simulink model "project_bonus"  (R2012b)
settings: Solver=ode45  StartTime=0.0  StopTime=Inf  FixedStep=0.01  RelTol=1e-3
libraries: simulink x2
settings Model: ExtModeTrigDuration=5000  Creator=adith  LastModifiedBy=adith
settings SolverCC: PositivePriorityOrder=on
settings RTWCC: SystemTargetFile=quarc_win64.tlc  TemplateMakefile=quarc_default_tmf  Description=QUARC Win64 Target  ProcessScript=quarc_win64_make_rtw_hook
settings STFCustomTargetCC: TargetPreCompLibLocation=C:\PROGRA~3\QUARC\lib\2012b\win64\release  CodeReplacementLibrary=ANSI_C  GeneratePreprocessorConditionals=Disable all  CombineOutputUpdateFcns=on  GRTInterface=off  SystemTargetFile=quarc_win64.tlc
settings GRTTargetCC: TargetPreCompLibLocation=C:\PROGRA~3\QUARC\lib\2012b\win64\release  ParMdlRefBuildCompliant=off  CompOptLevelCompliant=off  ConcurrentExecutionCompliant=off  MatFileLogging=off  ExtMode=on  ExtModeMexFile=quarc_comm

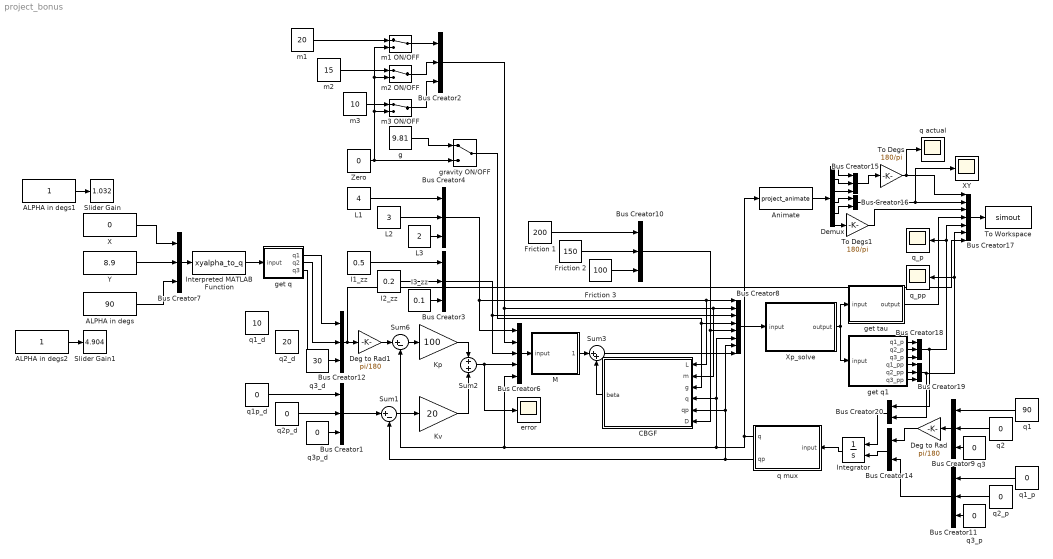
== system project_bonus ==
  ALPHA in degs : Constant  Value=90
  ALPHA in degs1 : Constant
  ALPHA in degs2 : Constant
  Animate : MATLABFcn  MATLABFcn=project_animate  OutputDimensions=6  OutputSignalType=real
  Bus Creator{1..4,7,9..12,15,18..19} (12 alike) : BusCreator  Inputs=3
  Bus Creator14 : BusCreator  Inputs=2
  Bus Creator16 : BusCreator  Inputs=2
  Bus Creator17 : BusCreator  Inputs=7
  Bus Creator20 : BusCreator  Inputs=2
  Bus Creator6 : BusCreator  Inputs=5
  Bus Creator8 : BusCreator  Inputs=8
  CBGF : MATLAB Function  TreatAsAtomicUnit=on
  Deg to Rad : Gain  Gain=pi/180
  Deg to Rad1 : Gain  Gain=pi/180
  Demux : Demux  Outputs=6
  Friction 1 : Constant  Value=200
  Friction 2 : Constant  Value=150
  Friction 3 : Constant  Value=100
  I1_zz : Constant  Value=0.5
  I2_zz : Constant  Value=0.2
  I3_zz : Constant  Value=0.1
  Integrator : Integrator  InitialConditionSource=external
  Interpreted MATLAB Function : MATLABFcn  MATLABFcn=xyalpha_to_q  OutputDimensions=3
  Kp : Gain  Gain=100
  Kv : Gain  Gain=20
  L1 : Constant  Value=4
  L2 : Constant  Value=3
  L3 : Constant  Value=2
  M : MATLAB Function  TreatAsAtomicUnit=on
  Slider Gain : simulink/Math Operations/Slider Gain  low=-4  gain=1.032  high=8.9
  Slider Gain1 : simulink/Math Operations/Slider Gain  low=3.5  gain=4.904  high=8.9
  Sum1 : Sum  Inputs=|+-
  Sum2 : Sum  Inputs=+|+
  Sum3 : Sum  Inputs=|++
  Sum6 : Sum  Inputs=|+-
  To Degs : Gain  Gain=180/pi
  To Degs1 : Gain  Gain=180/pi
  To Workspace : ToWorkspace  VariableName=simout  SampleTime=-1  SaveFormat=Structure With Time
  X : Constant  Value=0
  XY : Scope
      settings: ShowLegends=on  TimeRange=10  YMin=-8  YMax=9  SaveName=ScopeData4
  Xp_solve : MATLAB Function  TreatAsAtomicUnit=on
  Y : Constant  Value=8.9
  Zero : Constant  Value=0
  error : Scope
      settings: ShowLegends=on  TimeRange=8  YMin=-2.75  YMax=2.5  SaveName=ScopeData3
  g : Constant  Value=9.81
  get q : MATLAB Function  TreatAsAtomicUnit=on
  get q1 : MATLAB Function  TreatAsAtomicUnit=on
  get tau : MATLAB Function  TreatAsAtomicUnit=on
  gravity ON/OFF : ManualSwitch
  m1 : Constant  Value=20
  m1 ON/OFF : ManualSwitch
  m2 : Constant  Value=15
  m2 ON/OFF : ManualSwitch
  m3 : Constant  Value=10
  m3 ON/OFF : ManualSwitch
  q actual : Scope
      settings: ShowLegends=on  TimeRange=10  YMin=-100  YMax=175
  q mux : MATLAB Function  TreatAsAtomicUnit=on
  q1 : Constant  Value=90
  q1_d : Constant  Value=10
  q1_p : Constant  Value=0
  q1p_d : Constant  Value=0
  q2 : Constant  Value=0
  q2_d : Constant  Value=20
  q2_p : Constant  Value=0
  q2p_d : Constant  Value=0
  q3 : Constant  Value=0
  q3_d : Constant  Value=30
  q3_p : Constant  Value=0
  q3p_d : Constant  Value=0
  q_p : Scope
      settings: ShowLegends=on  TimeRange=20  YMin=-1.75  YMax=1.5
  q_pp : Scope
      settings: ShowLegends=on  TimeRange=20  YMin=-75  YMax=40  SaveName=ScopeData2
  wires:
  Bus Creator7/1 -> Interpreted MATLAB Function/1
  Interpreted MATLAB Function/1 -> get q/1(input)
  ALPHA in degs1/1 -> Slider Gain/1
  m1/1 -> m1 ON/OFF/1
  m3 ON/OFF/1 -> Bus Creator2/3
  m3/1 -> m3 ON/OFF/1
  m1 ON/OFF/1 -> Bus Creator2/1
  m2 ON/OFF/1 -> Bus Creator2/2
  m2/1 -> m2 ON/OFF/1
  Zero/1 -> m1 ON/OFF/2, m2 ON/OFF/2, m3 ON/OFF/2, gravity ON/OFF/2
  Friction 3/1 -> Bus Creator10/3
  Friction 2/1 -> Bus Creator10/2
  Friction 1/1 -> Bus Creator10/1
  g/1 -> gravity ON/OFF/1
  q1p_d/1 -> Bus Creator1/1
  q2p_d/1 -> Bus Creator1/2
  q3p_d/1 -> Bus Creator1/3
  I2_zz/1 -> Bus Creator3/2
  I3_zz/1 -> Bus Creator3/3
  L1/1 -> Bus Creator4/1
  L2/1 -> Bus Creator4/2
  L3/1 -> Bus Creator4/3
  Sum6/1 -> Kp/1
  Sum1/1 -> Kv/1
  Bus Creator1/1 -> Sum1/1
  Kp/1 -> Sum2/1
  Kv/1 -> Sum2/2
  Bus Creator4/1 -> CBGF/1(L), Bus Creator8/1, Bus Creator6/1
  Bus Creator2/1 -> CBGF/2(m), Bus Creator8/2, Bus Creator6/2
  Bus Creator3/1 -> Bus Creator6/3, Bus Creator8/3
  Sum2/1 -> error/1, Bus Creator6/4
  Bus Creator6/1 -> M/1(input)
  M/1(tau_wM) -> Sum3/1
  CBGF/1(beta) -> Sum3/2
  gravity ON/OFF/1 -> CBGF/3(g), Bus Creator8/4
  Bus Creator10/1 -> CBGF/6(D), Bus Creator8/5
  I1_zz/1 -> Bus Creator3/1
  Sum3/1 -> Bus Creator8/8
  Integrator/1 -> q mux/1(input)
  Bus Creator8/1 -> Xp_solve/1(input)
  q1/1 -> Bus Creator9/1
  q2/1 -> Bus Creator9/2
  q3/1 -> Bus Creator9/3
  q1_p/1 -> Bus Creator11/1
  q2_p/1 -> Bus Creator11/2
  q3_p/1 -> Bus Creator11/3
  Bus Creator11/1 -> Bus Creator14/2
  Bus Creator9/1 -> Deg to Rad/1
  Deg to Rad/1 -> Bus Creator14/1
  Bus Creator12/1 -> Bus Creator17/7, Deg to Rad1/1
  Deg to Rad1/1 -> Sum6/1
  q mux/1(q) -> Bus Creator8/6, CBGF/4(q), Bus Creator6/5, Sum6/2, Animate/1
  q mux/2(qp) -> Bus Creator8/7, CBGF/5(qp), Sum1/2
  Bus Creator17/1 -> To Workspace/1
  Animate/1 -> Demux/1
  Demux/1 -> Bus Creator15/1
  Demux/2 -> Bus Creator15/2
  Demux/3 -> Bus Creator15/3
  Bus Creator15/1 -> To Degs/1
  Demux/4 -> Bus Creator16/1
  Demux/5 -> Bus Creator16/2
  Demux/6 -> To Degs1/1
  To Degs/1 -> q actual/1, Bus Creator17/1
  Bus Creator16/1 -> XY/1, Bus Creator17/2
  To Degs1/1 -> Bus Creator17/3
  Xp_solve/1(output) -> get q1/1(input), get tau/1(input)
  get tau/1(output) -> Bus Creator17/4
  Bus Creator18/1 -> Bus Creator20/1, q_p/1, Bus Creator17/5
  Bus Creator19/1 -> Bus Creator20/2, q_pp/1, Bus Creator17/6
  Bus Creator20/1 -> Integrator/1
  get q1/1(q1_p) -> Bus Creator18/1
  get q1/2(q2_p) -> Bus Creator18/2
  get q1/3(q3_p) -> Bus Creator18/3
  get q1/4(q1_pp) -> Bus Creator19/1
  get q1/5(q2_pp) -> Bus Creator19/2
  get q1/6(q3_pp) -> Bus Creator19/3
  get q/1(q1) -> Bus Creator12/1
  get q/2(q2) -> Bus Creator12/2
  get q/3(q3) -> Bus Creator12/3
  Bus Creator14/1 -> Integrator/2
  ALPHA in degs2/1 -> Slider Gain1/1
  ALPHA in degs/1 -> Bus Creator7/3
  X/1 -> Bus Creator7/1
  Y/1 -> Bus Creator7/2

== matlab function project_bonus/M ==
  data: input input; tau_wM output
function tau_wM  = M_matrix(input)
    L1 = input(1);
    L2 = input(2);
    L3 = input(3);
    m1 = input(4);
    m2 = input(5);
    m3 = input(6);
    I1_zz = input(7);
    I2_zz = input(8);
    I3_zz = input(9);
    tau1 = input(10);
    tau2 = input(11);
    tau3 = input(12);
    q1 = input(13);
    q2 = input(14);
    q3 = input(15);
%     g = input(10);
%     D1 = input(11);
%     D2 = input(12);
%     D3 = input(13);
    tau_p = [tau1; tau2; tau3];
    M = [(I1_zz + I2_zz + I3_zz + (L1^2*m1)/4 + L1^2*m2 + L1^2*m3 + (L2^2*m2)/4 + L2^2*m3 + (L3^2*m3)/4 + L1*L3*m3*cos(q2 + q3) + L1*L2*m2*cos(q2) + 2*L1*L2*m3*cos(q2) + L2*L3*m3*cos(q3)), (I2_zz + I3_zz + (L2^2*m2)/4 + L2^2*m3 + (L3^2*m3)/4 + (L1*L3*m3*cos(q2 + q3))/2 + (L1*L2*m2*cos(q2))/2 + L1*L2*m3*cos(q2) + L2*L3*m3*cos(q3)), (I3_zz + (L3^2*m3)/4 + (L1*L3*m3*cos(q2 + q3))/2 + (L2*L3*m3*cos(q3))/2);
         (I2_zz + I3_zz + (L2^2*m2)/4 + L2^2*m3 + (L3^2*m3)/4 + (L1*L3*m3*cos(q2 + q3))/2 + (L1*L2*m2*cos(q2))/2 + L1*L2*m3*cos(q2) + L2*L3*m3*cos(q3)),                                                                       (I2_zz + I3_zz + (L2^2*m2)/4 + L2^2*m3 + (L3^2*m3)/4 + L2*L3*m3*cos(q3)),                             ((m3*L3^2)/4 + (L2*m3*cos(q3)*L3)/2 + I3_zz);
         (I3_zz + (L3^2*m3)/4 + (L1*L3*m3*cos(q2 + q3))/2 + (L2*L3*m3*cos(q3))/2),                                                                                                   ((m3*L3^2)/4 + (L2*m3*cos(q3)*L3)/2 + I3_zz),                                                    ((m3*L3^2)/4 + I3_zz)];
    tau_wM = M*tau_p;
end

== matlab function project_bonus/CBGF ==
  data: L input; beta output; m input; g input; q input; qp input; D input
function beta  = CBGF(L, m, g, q, qp, D)
    L1 = L(1);
    L2 = L(2);
    L3 = L(3);
    m1 = m(1);
    m2 = m(2);
    m3 = m(3);
    q1 = q(1);
    q2 = q(2);
    q3 = q(3);
    q1_p = qp(1);
    q2_p = qp(2);
    q3_p = qp(3);
    D1 = D(1);
    D2 = D(2);
    D3 = D(3);
        
%     g = input(10);
%     D1 = input(11);
%     D2 = input(12);
%     D3 = input(13);

    G =[((5*g*(7*L2*cos(q1 + q2) + 14*L1*cos(q1) + 2*L3*cos(q1 + q2 + q3)))/2);
                  (5*L3*g*cos(q1 + q2 + q3) + (35*L2*g*cos(q1 + q2))/2);
                                             (5*L3*g*cos(q1 + q2 + q3))]; 
    F = [D1*q1_p;
        D2*q2_p;
        D3*q3_p];
    B = [ (-L1*(L3*m3*sin(q2 + q3) + L2*m2*sin(q2) + 2*L2*m3*sin(q2))), (-L3*m3*(L1*sin(q2 + q3) + L2*sin(q3))), (-L3*m3*(L1*sin(q2 + q3) + L2*sin(q3)));
                                                          0,                     (-L2*L3*m3*sin(q3)),                     (-L2*L3*m3*sin(q3));
                                           (L2*L3*m3*sin(q3)),                                     0,                                     0];

    C =[                                                             0, (-(L1*(L3*m3*sin(q2 + q3) + L2*m2*sin(q2) + 2*L2*m3*sin(q2)))/2), (-(L3*m3*(L1*sin(q2 + q3) + L2*sin(q3)))/2);
         ((L1*(L3*m3*sin(q2 + q3) + L2*m2*sin(q2) + 2*L2*m3*sin(q2)))/2),                                                              0,                     (-(L2*L3*m3*sin(q3))/2);
                              ((L3*m3*(L1*sin(q2 + q3) + L2*sin(q3)))/2),                                           ((L2*L3*m3*sin(q3))/2),                                         0];
    V =  C*[q1_p^2; q2_p^2; q3_p^2] + B*[q1_p*q2_p; q1_p*q3_p; q2_p*q3_p];
    beta = V + G + F;
end

== matlab function project_bonus/get tau ==
  data: input input; output output
function output  = get_tau(input)
    tau1 = input(7);
    tau2 = input(8);
    tau3 = input(9);
    output = [tau1, tau2, tau3];
end

== matlab function project_bonus/get q ==
  data: input input; q1 output; q2 output; q3 output
function [q1, q2, q3]  = get_q(input)
    q1 = input(1);
    q2 = input(2);
    q3 = input(3);
%     q1 = atan2(sin(q1),cos(q1));
%     q2 = atan2(sin(q2),cos(q2));
%     q3 = atan2(sin(q3),cos(q3));
    %output = [q1, q2, q3, q1_p, q2_p, q3_p];
end

== matlab function project_bonus/get q1 ==
  data: input input; q1_p output; q2_p output; q3_p output; q1_pp output; q2_pp output; q3_pp output
function [q1_p, q2_p, q3_p, q1_pp, q2_pp, q3_pp]  = get_q(input)
    q1_p = input(1);
    q2_p = input(2);
    q3_p = input(3);
    q1_pp = input(4);
    q2_pp = input(5);
    q3_pp = input(6);
    %output = [q1_p, q2_p, q3_p, q1_pp, q2_pp, q3_pp];
end

== matlab function project_bonus/Xp_solve ==
  data: input input; output output
function output  = Xp_solve(input)
    L1 = input(1);
    L2 = input(2);
    L3 = input(3);
    m1 = input(4);
    m2 = input(5);
    m3 = input(6);
    I1_zz = input(7);
    I2_zz = input(8);
    I3_zz = input(9);
    g = input(10);
    D1 = input(11);
    D2 = input(12);
    D3 = input(13);
    q1 = input(14);
    q2 = input(15);
    q3 = input(16);
    q1_p = input(17);
    q2_p = input(18);
    q3_p = input(19);
    tau1 = input(20);
    tau2 = input(21);
    tau3 = input(22);
    q1_pp = (2*(32*I2_zz*I3_zz*tau1 - 32*I2_zz*I3_zz*tau2 + 8*I3_zz*L2^2*m2*tau1 + 8*I2_zz*L3^2*m3*tau1 - 8*I3_zz*L2^2*m2*tau2 + 32*I3_zz*L2^2*m3*tau1 - 8*I2_zz*L3^2*m3*tau2 - 32*I3_zz*L2^2*m3*tau2 - 32*D1*I2_zz*I3_zz*q1_p + 32*D2*I2_zz*I3_zz*q2_p + 4*L2^2*L3^2*m3^2*tau1 - 4*L2^2*L3^2*m3^2*tau2 + 2*L2^2*L3^2*m2*m3*tau1 - 2*L2^2*L3^2*m2*m3*tau2 - 4*L2^2*L3^2*m3^2*tau1*cos(2*q3) + 4*L2^2*L3^2*m3^2*tau2*cos(2*q3) - 4*D1*L2^2*L3^2*m3^2*q1_p + 4*D2*L2^2*L3^2*m3^2*q2_p - 8*D1*I3_zz*L2^2*m2*q1_p - 8*D1*I2_zz*L3^2*m3*q1_p - 32*D1*I3_zz*L2^2*m3*q1_p + 8*D2*I3_zz*L2^2*m2*q2_p + 8*D2*I2_zz*L3^2*m3*q2_p + 32*D2*I3_zz*L2^2*m3*q2_p - 1120*I2_zz*I3_zz*L1*g*cos(q1) - 85*L1*L2^2*L3^2*g*m3^2*cos(q1) - 15*L1*L2^2*L3^2*g*m3^2*cos(q1 + 2*q2 + 2*q3) + 4*I2_zz*L1^2*L3^2*m3^2*q1_p^2*sin(2*q2 + 2*q3) + 4*I3_zz*L1*L2^3*m2^2*q1_p^2*sin(q2) + 4*I3_zz*L1*L2^3*m2^2*q2_p^2*sin(q2) + 32*I3_zz*L1*L2^3*m3^2*q1_p^2*sin(q2) + 32*I3_zz*L1*L2^3*m3^2*q2_p^2*sin(q2) + 15*L1*L2^2*L3^2*g*m3^2*cos(q1 + 2*q2) + 35*L1*L2^2*L3^2*g*m3^2*cos(q1 - 2*q3) + 50*L1*L2^2*L3^2*g*m3^2*cos(q1 + 2*q3) - 2*D1*L2^2*L3^2*m2*m3*q1_p + 2*D2*L2^2*L3^2*m2*m3*q2_p - 140*I3_zz*L1*L2^2*g*m2*cos(q1) - 240*I2_zz*L1*L3^2*g*m3*cos(q1) - 840*I3_zz*L1*L2^2*g*m3*cos(q1) + 40*I2_zz*L1*L3^2*g*m3*cos(q1 + 2*q2 + 2*q3) + 4*D1*L2^2*L3^2*m3^2*q1_p*cos(2*q3) - 4*D2*L2^2*L3^2*m3^2*q2_p*cos(2*q3) + 140*I3_zz*L1*L2^2*g*m2*cos(q1 + 2*q2) + 280*I3_zz*L1*L2^2*g*m3*cos(q1 + 2*q2) - 8*L1*L2^2*L3*m3^2*tau3*cos(q2 + q3) - 4*L1*L2*L3^2*m3^2*tau2*cos(q2) + 4*L1*L2*L3^2*m3^2*tau3*cos(q2) - 16*I2_zz*L1*L3*m3*tau3*cos(q2 + q3) + 4*I3_zz*L1^2*L2^2*m2^2*q1_p^2*sin(2*q2) + 16*I3_zz*L1^2*L2^2*m3^2*q1_p^2*sin(2*q2) + 4*L1*L2*L3^2*m3^2*tau2*cos(q2 + 2*q3) + 8*L1*L2^2*L3*m3^2*tau3*cos(q2 - q3) - 4*L1*L2*L3^2*m3^2*tau3*cos(q2 + 2*q3) + 4*I2_zz*L1*L3^3*m3^2*q1_p^2*sin(q2 + q3) + 4*I2_zz*L1*L3^3*m3^2*q2_p^2*sin(q2 + q3) + 4*I2_zz*L1*L3^3*m3^2*q3_p^2*sin(q2 + q3) - 16*I3_zz*L1*L2*m2*tau2*cos(q2) + 16*I3_zz*L1*L2*m2*tau3*cos(q2) - 32*I3_zz*L1*L2*m3*tau2*cos(q2) + 32*I3_zz*L1*L2*m3*tau3*cos(q2) + 8*I2_zz*L1*L3^3*m3^2*q1_p*q2_p*sin(q2 + q3) + 8*I2_zz*L1*L3^3*m3^2*q1_p*q3_p*sin(q2 + q3) + 8*I2_zz*L1*L3^3*m3^2*q2_p*q3_p*sin(q2 + q3) + 16*D3*I2_zz*L1*L3*m3*q3_p*cos(q2 + q3) - 35*L1*L2^2*L3^2*g*m2*m3*cos(q1) + L1*L2^2*L3^3*m2*m3^2*q1_p^2*sin(q2 - q3) + L1*L2^2*L3^3*m2*m3^2*q2_p^2*sin(q2 - q3) - L1*L2^3*L3^2*m2*m3^2*q1_p^2*sin(q2 + 2*q3) + L1*L2^2*L3^3*m2*m3^2*q3_p^2*sin(q2 - q3) - L1*L2^3*L3^2*m2*m3^2*q2_p^2*sin(q2 + 2*q3) - 4*D2*L1*L2*L3^2*m3^2*q2_p*cos(q2 + 2*q3) - 8*D3*L1*L2^2*L3*m3^2*q3_p*cos(q2 - q3) + 4*D3*L1*L2*L3^2*m3^2*q3_p*cos(q2 + 2*q3) + 24*I3_zz*L1*L2^3*m2*m3*q1_p^2*sin(q2) + 24*I3_zz*L1*L2^3*m2*m3*q2_p^2*sin(q2) + 8*I3_zz*L1*L2^3*m2^2*q1_p*q2_p*sin(q2) + 64*I3_zz*L1*L2^3*m3^2*q1_p*q2_p*sin(q2) + 16*D2*I3_zz*L1*L2*m2*q2_p*cos(q2) + 32*D2*I3_zz*L1*L2*m3*q2_p*cos(q2) - 16*D3*I3_zz*L1*L2*m2*q3_p*cos(q2) - 32*D3*I3_zz*L1*L2*m3*q3_p*cos(q2) + 8*I3_zz*L1*L2^2*L3*m3^2*q1_p^2*sin(q2 + q3) + 8*I3_zz*L1*L2^2*L3*m3^2*q2_p^2*sin(q2 + q3) + 8*I3_zz*L1*L2^2*L3*m3^2*q3_p^2*sin(q2 + q3) + 25*L1*L2^2*L3^2*g*m2*m3*cos(q1 + 2*q2) - 10*L1*L2^2*L3^2*g*m2*m3*cos(q1 + 2*q3) + 4*I2_zz*L1*L2*L3^2*m3^2*q1_p^2*sin(q2) + 4*I2_zz*L1*L2*L3^2*m3^2*q2_p^2*sin(q2) + 16*I2_zz*I3_zz*L1*L3*m3*q1_p^2*sin(q2 + q3) + 16*I2_zz*I3_zz*L1*L3*m3*q2_p^2*sin(q2 + q3) + 16*I2_zz*I3_zz*L1*L3*m3*q3_p^2*sin(q2 + q3) + 4*I2_zz*L1*L2*L3^2*m3^2*q1_p^2*sin(q2 + 2*q3) + 8*I3_zz*L1*L2^2*L3*m3^2*q1_p^2*sin(q2 - q3) + 4*I2_zz*L1*L2*L3^2*m3^2*q2_p^2*sin(q2 + 2*q3) + 8*I3_zz*L1*L2^2*L3*m3^2*q2_p^2*sin(q2 - q3) + 8*I3_zz*L1*L2^2*L3*m3^2*q3_p^2*sin(q2 - q3) + 16*I2_zz*I3_zz*L1*L2*m2*q1_p^2*sin(q2) + 16*I2_zz*I3_zz*L1*L2*m2*q2_p^2*sin(q2) + 32*I2_zz*I3_zz*L1*L2*m3*q1_p^2*sin(q2) + 32*I2_zz*I3_zz*L1*L2*m3*q2_p^2*sin(q2) + 2*L1^2*L2^2*L3^2*m2*m3^2*q1_p^2*sin(2*q2) + L1^2*L2^2*L3^2*m2^2*m3*q1_p^2*sin(2*q2) - 4*L1*L2*L3^2*m2*m3*tau2*cos(q2) + 4*L1*L2*L3^2*m2*m3*tau3*cos(q2) + 8*D3*L1*L2^2*L3*m3^2*q3_p*cos(q2 + q3) - L1^2*L2^2*L3^2*m2*m3^2*q1_p^2*sin(2*q2 + 2*q3) + 16*I3_zz*L1^2*L2^2*m2*m3*q1_p^2*sin(2*q2) + 3*L1*L2^3*L3^2*m2*m3^2*q1_p^2*sin(q2) + L1*L2^3*L3^2*m2^2*m3*q1_p^2*sin(q2) + 3*L1*L2^3*L3^2*m2*m3^2*q2_p^2*sin(q2) + L1*L2^3*L3^2*m2^2*m3*q2_p^2*sin(q2) + 4*L1*L2^2*L3*m2*m3*tau3*cos(q2 - q3) + 4*D2*L1*L2*L3^2*m3^2*q2_p*cos(q2) - 4*D3*L1*L2*L3^2*m3^2*q3_p*cos(q2) + 6*L1*L2^3*L3^2*m2*m3^2*q1_p*q2_p*sin(q2) + 2*L1*L2^3*L3^2*m2^2*m3*q1_p*q2_p*sin(q2) + 4*D2*L1*L2*L3^2*m2*m3*q2_p*cos(q2) - 4*D3*L1*L2*L3^2*m2*m3*q3_p*cos(q2) + 2*L1*L2^2*L3^3*m2*m3^2*q1_p*q2_p*sin(q2 - q3) + 2*L1*L2^2*L3^3*m2*m3^2*q1_p*q3_p*sin(q2 - q3) - 2*L1*L2^3*L3^2*m2*m3^2*q1_p*q2_p*sin(q2 + 2*q3) + 2*L1*L2^2*L3^3*m2*m3^2*q2_p*q3_p*sin(q2 - q3) - 4*D3*L1*L2^2*L3*m2*m3*q3_p*cos(q2 - q3) + 48*I3_zz*L1*L2^3*m2*m3*q1_p*q2_p*sin(q2) + 16*I3_zz*L1*L2^2*L3*m3^2*q1_p*q2_p*sin(q2 + q3) + 16*I3_zz*L1*L2^2*L3*m3^2*q1_p*q3_p*sin(q2 + q3) + 16*I3_zz*L1*L2^2*L3*m3^2*q2_p*q3_p*sin(q2 + q3) + 4*I2_zz*L1*L2*L3^2*m2*m3*q1_p^2*sin(q2) + 4*I2_zz*L1*L2*L3^2*m2*m3*q2_p^2*sin(q2) + 8*I2_zz*L1*L2*L3^2*m3^2*q1_p*q2_p*sin(q2) + 32*I2_zz*I3_zz*L1*L3*m3*q1_p*q2_p*sin(q2 + q3) + 32*I2_zz*I3_zz*L1*L3*m3*q1_p*q3_p*sin(q2 + q3) + 32*I2_zz*I3_zz*L1*L3*m3*q2_p*q3_p*sin(q2 + q3) + 4*I3_zz*L1*L2^2*L3*m2*m3*q1_p^2*sin(q2 - q3) + 4*I3_zz*L1*L2^2*L3*m2*m3*q2_p^2*sin(q2 - q3) + 4*I3_zz*L1*L2^2*L3*m2*m3*q3_p^2*sin(q2 - q3) + 8*I2_zz*L1*L2*L3^2*m3^2*q1_p*q2_p*sin(q2 + 2*q3) + 16*I3_zz*L1*L2^2*L3*m3^2*q1_p*q2_p*sin(q2 - q3) + 16*I3_zz*L1*L2^2*L3*m3^2*q1_p*q3_p*sin(q2 - q3) + 16*I3_zz*L1*L2^2*L3*m3^2*q2_p*q3_p*sin(q2 - q3) + 32*I2_zz*I3_zz*L1*L2*m2*q1_p*q2_p*sin(q2) + 64*I2_zz*I3_zz*L1*L2*m3*q1_p*q2_p*sin(q2) + 8*I2_zz*L1*L2*L3^2*m2*m3*q1_p*q2_p*sin(q2) + 8*I3_zz*L1*L2^2*L3*m2*m3*q1_p*q2_p*sin(q2 - q3) + 8*I3_zz*L1*L2^2*L3*m2*m3*q1_p*q3_p*sin(q2 - q3) + 8*I3_zz*L1*L2^2*L3*m2*m3*q2_p*q3_p*sin(q2 - q3)))/(64*I1_zz*I2_zz*I3_zz + 16*I2_zz*I3_zz*L1^2*m1 + 16*I1_zz*I3_zz*L2^2*m2 + 64*I2_zz*I3_zz*L1^2*m2 + 16*I1_zz*I2_zz*L3^2*m3 + 64*I1_zz*I3_zz*L2^2*m3 + 64*I2_zz*I3_zz*L1^2*m3 + 8*I3_zz*L1^2*L2^2*m2^2 + 8*I1_zz*L2^2*L3^2*m3^2 + 8*I2_zz*L1^2*L3^2*m3^2 + 32*I3_zz*L1^2*L2^2*m3^2 - 8*I2_zz*L1^2*L3^2*m3^2*cos(2*q2 + 2*q3) + 2*L1^2*L2^2*L3^2*m1*m3^2 + 6*L1^2*L2^2*L3^2*m2*m3^2 + 2*L1^2*L2^2*L3^2*m2^2*m3 + 4*I3_zz*L1^2*L2^2*m1*m2 + 4*I2_zz*L1^2*L3^2*m1*m3 + 16*I3_zz*L1^2*L2^2*m1*m3 + 4*I1_zz*L2^2*L3^2*m2*m3 + 16*I2_zz*L1^2*L3^2*m2*m3 + 48*I3_zz*L1^2*L2^2*m2*m3 - 8*I3_zz*L1^2*L2^2*m2^2*cos(2*q2) - 32*I3_zz*L1^2*L2^2*m3^2*cos(2*q2) - 8*I1_zz*L2^2*L3^2*m3^2*cos(2*q3) - 32*I3_zz*L1^2*L2^2*m2*m3*cos(2*q2) + L1^2*L2^2*L3^2*m1*m2*m3 - 2*L1^2*L2^2*L3^2*m1*m3^2*cos(2*q3) - 4*L1^2*L2^2*L3^2*m2*m3^2*cos(2*q2) - 2*L1^2*L2^2*L3^2*m2^2*m3*cos(2*q2) - 4*L1^2*L2^2*L3^2*m2*m3^2*cos(2*q3) + 2*L1^2*L2^2*L3^2*m2*m3^2*cos(2*q2 + 2*q3)); 
    q2_pp = -(2*(32*I2_zz*I3_zz*tau1 - 32*I1_zz*I3_zz*tau2 + 32*I1_zz*I3_zz*tau3 - 32*I2_zz*I3_zz*tau2 - 8*I3_zz*L1^2*m1*tau2 + 8*I3_zz*L1^2*m1*tau3 - 32*I3_zz*L1^2*m2*tau2 + 8*I3_zz*L2^2*m2*tau1 - 8*I1_zz*L3^2*m3*tau2 + 8*I2_zz*L3^2*m3*tau1 + 32*I3_zz*L1^2*m2*tau3 - 32*I3_zz*L1^2*m3*tau2 - 8*I3_zz*L2^2*m2*tau2 + 32*I3_zz*L2^2*m3*tau1 + 8*I1_zz*L3^2*m3*tau3 - 8*I2_zz*L3^2*m3*tau2 + 32*I3_zz*L1^2*m3*tau3 - 32*I3_zz*L2^2*m3*tau2 - 32*D1*I2_zz*I3_zz*q1_p + 32*D2*I1_zz*I3_zz*q2_p + 32*D2*I2_zz*I3_zz*q2_p - 32*D3*I1_zz*I3_zz*q3_p - 4*L1^2*L3^2*m3^2*tau2 + 4*L2^2*L3^2*m3^2*tau1 + 4*L1^2*L3^2*m3^2*tau3 - 4*L2^2*L3^2*m3^2*tau2 - 2*L1^2*L3^2*m1*m3*tau2 + 2*L1^2*L3^2*m1*m3*tau3 - 8*L1^2*L3^2*m2*m3*tau2 + 2*L2^2*L3^2*m2*m3*tau1 + 8*L1^2*L3^2*m2*m3*tau3 - 2*L2^2*L3^2*m2*m3*tau2 - 4*L2^2*L3^2*m3^2*tau1*cos(2*q3) + 4*L2^2*L3^2*m3^2*tau2*cos(2*q3) - 4*D1*L2^2*L3^2*m3^2*q1_p + 4*D2*L1^2*L3^2*m3^2*q2_p + 4*D2*L2^2*L3^2*m3^2*q2_p - 4*D3*L1^2*L3^2*m3^2*q3_p + 560*I1_zz*I3_zz*L2*g*cos(q1 + q2) + 4*L1^2*L3^2*m3^2*tau2*cos(2*q2 + 2*q3) - 4*L1^2*L3^2*m3^2*tau3*cos(2*q2 + 2*q3) - 8*D1*I3_zz*L2^2*m2*q1_p + 8*D2*I3_zz*L1^2*m1*q2_p - 8*D1*I2_zz*L3^2*m3*q1_p - 32*D1*I3_zz*L2^2*m3*q1_p + 32*D2*I3_zz*L1^2*m2*q2_p + 8*D2*I1_zz*L3^2*m3*q2_p + 32*D2*I3_zz*L1^2*m3*q2_p + 8*D2*I3_zz*L2^2*m2*q2_p - 8*D3*I3_zz*L1^2*m1*q3_p + 8*D2*I2_zz*L3^2*m3*q2_p + 32*D2*I3_zz*L2^2*m3*q2_p - 32*D3*I3_zz*L1^2*m2*q3_p - 8*D3*I1_zz*L3^2*m3*q3_p - 32*D3*I3_zz*L1^2*m3*q3_p - 1120*I2_zz*I3_zz*L1*g*cos(q1) - 85*L1*L2^2*L3^2*g*m3^2*cos(q1) + 35*L1^2*L2*L3^2*g*m3^2*cos(q1 - q2 - 2*q3) - 15*L1*L2^2*L3^2*g*m3^2*cos(q1 + 2*q2 + 2*q3) - 15*L1^2*L2*L3^2*g*m3^2*cos(q1 + 3*q2 + 2*q3) + 4*I2_zz*L1^2*L3^2*m3^2*q1_p^2*sin(2*q2 + 2*q3) + 140*I3_zz*L1^2*L2*g*m1*cos(q1 + q2) + 280*I3_zz*L1^2*L2*g*m2*cos(q1 + q2) + 100*I1_zz*L2*L3^2*g*m3*cos(q1 + q2) + 4*I3_zz*L1*L2^3*m2^2*q1_p^2*sin(q2) + 16*I3_zz*L1^3*L2*m2^2*q1_p^2*sin(q2) + 4*I3_zz*L1*L2^3*m2^2*q2_p^2*sin(q2) + 32*I3_zz*L1*L2^3*m3^2*q1_p^2*sin(q2) + 32*I3_zz*L1^3*L2*m3^2*q1_p^2*sin(q2) - 4*I1_zz*L2*L3^3*m3^2*q1_p^2*sin(q3) + 32*I3_zz*L1*L2^3*m3^2*q2_p^2*sin(q2) - 4*I1_zz*L2*L3^3*m3^2*q2_p^2*sin(q3) - 4*I1_zz*L2*L3^3*m3^2*q3_p^2*sin(q3) - 50*L1^2*L2*L3^2*g*m3^2*cos(q1 - q2) + 15*L1*L2^2*L3^2*g*m3^2*cos(q1 + 2*q2) + 35*L1*L2^2*L3^2*g*m3^2*cos(q1 - 2*q3) + 50*L1*L2^2*L3^2*g*m3^2*cos(q1 + 2*q3) - 2*D1*L2^2*L3^2*m2*m3*q1_p + 2*D2*L1^2*L3^2*m1*m3*q2_p + 8*D2*L1^2*L3^2*m2*m3*q2_p + 2*D2*L2^2*L3^2*m2*m3*q2_p - 2*D3*L1^2*L3^2*m1*m3*q3_p - 8*D3*L1^2*L3^2*m2*m3*q3_p - 140*I3_zz*L1*L2^2*g*m2*cos(q1) - 240*I2_zz*L1*L3^2*g*m3*cos(q1) - 840*I3_zz*L1*L2^2*g*m3*cos(q1) + 40*I2_zz*L1*L3^2*g*m3*cos(q1 + 2*q2 + 2*q3) + 4*D1*L2^2*L3^2*m3^2*q1_p*cos(2*q3) - 4*D2*L2^2*L3^2*m3^2*q2_p*cos(2*q3) - 280*I3_zz*L1^2*L2*g*m2*cos(q1 - q2) + 140*I3_zz*L1*L2^2*g*m2*cos(q1 + 2*q2) - 560*I3_zz*L1^2*L2*g*m3*cos(q1 - q2) + 280*I3_zz*L1*L2^2*g*m3*cos(q1 + 2*q2) - 8*L1*L2^2*L3*m3^2*tau3*cos(q2 + q3) - 4*D2*L1^2*L3^2*m3^2*q2_p*cos(2*q2 + 2*q3) + 4*D3*L1^2*L3^2*m3^2*q3_p*cos(2*q2 + 2*q3) + 50*L1^2*L2*L3^2*g*m3^2*cos(q1 + q2 + 2*q3) + 4*L1*L2*L3^2*m3^2*tau1*cos(q2) - 8*L1*L2*L3^2*m3^2*tau2*cos(q2) + 4*L1*L2*L3^2*m3^2*tau3*cos(q2) + 8*L1^2*L2*L3*m3^2*tau3*cos(q3) - 16*I2_zz*L1*L3*m3*tau3*cos(q2 + q3) - 20*L1^2*L2*L3^2*g*m3^2*cos(q1 + q2) + 8*I3_zz*L1^2*L2^2*m2^2*q1_p^2*sin(2*q2) + 4*I3_zz*L1^2*L2^2*m2^2*q2_p^2*sin(2*q2) + 32*I3_zz*L1^2*L2^2*m3^2*q1_p^2*sin(2*q2) - 4*I1_zz*L2^2*L3^2*m3^2*q1_p^2*sin(2*q3) + 16*I3_zz*L1^2*L2^2*m3^2*q2_p^2*sin(2*q2) - 4*I1_zz*L2^2*L3^2*m3^2*q2_p^2*sin(2*q3) - 4*L1*L2*L3^2*m3^2*tau1*cos(q2 + 2*q3) + 8*L1*L2*L3^2*m3^2*tau2*cos(q2 + 2*q3) + 8*L1*L2^2*L3*m3^2*tau3*cos(q2 - q3) - 4*L1*L2*L3^2*m3^2*tau3*cos(q2 + 2*q3) - 8*L1^2*L2*L3*m3^2*tau3*cos(2*q2 + q3) - 40*I1_zz*L2*L3^2*g*m3*cos(q1 + q2 + 2*q3) + 4*I2_zz*L1*L3^3*m3^2*q1_p^2*sin(q2 + q3) + 4*I2_zz*L1*L3^3*m3^2*q2_p^2*sin(q2 + q3) + 4*I2_zz*L1*L3^3*m3^2*q3_p^2*sin(q2 + q3) + 16*I3_zz*L1*L2*m2*tau1*cos(q2) - 32*I3_zz*L1*L2*m2*tau2*cos(q2) + 32*I3_zz*L1*L2*m3*tau1*cos(q2) + 16*I3_zz*L1*L2*m2*tau3*cos(q2) - 64*I3_zz*L1*L2*m3*tau2*cos(q2) + 32*I3_zz*L1*L2*m3*tau3*cos(q2) + 16*I1_zz*L2*L3*m3*tau3*cos(q3) + 8*I2_zz*L1*L3^3*m3^2*q1_p*q2_p*sin(q2 + q3) + 8*I2_zz*L1*L3^3*m3^2*q1_p*q3_p*sin(q2 + q3) + 8*I2_zz*L1*L3^3*m3^2*q2_p*q3_p*sin(q2 + q3) + 16*D3*I2_zz*L1*L3*m3*q3_p*cos(q2 + q3) - 35*L1*L2^2*L3^2*g*m2*m3*cos(q1) + 10*L1^2*L2*L3^2*g*m2*m3*cos(q1 + 3*q2 + 2*q3) + L1*L2^2*L3^3*m2*m3^2*q1_p^2*sin(q2 - q3) - L1^3*L2*L3^2*m1*m3^2*q1_p^2*sin(q2 + 2*q3) + L1*L2^2*L3^3*m2*m3^2*q2_p^2*sin(q2 - q3) - L1*L2^3*L3^2*m2*m3^2*q1_p^2*sin(q2 + 2*q3) + L1^2*L2*L3^3*m2*m3^2*q1_p^2*sin(2*q2 + q3) - 2*L1^3*L2*L3^2*m2*m3^2*q1_p^2*sin(q2 + 2*q3) + L1*L2^2*L3^3*m2*m3^2*q3_p^2*sin(q2 - q3) - L1*L2^3*L3^2*m2*m3^2*q2_p^2*sin(q2 + 2*q3) + L1^2*L2*L3^3*m2*m3^2*q2_p^2*sin(2*q2 + q3) + L1^2*L2*L3^3*m2*m3^2*q3_p^2*sin(2*q2 + q3) + 4*D1*L1*L2*L3^2*m3^2*q1_p*cos(q2 + 2*q3) - 8*D2*L1*L2*L3^2*m3^2*q2_p*cos(q2 + 2*q3) - 8*D3*L1*L2^2*L3*m3^2*q3_p*cos(q2 - q3) + 4*D3*L1*L2*L3^2*m3^2*q3_p*cos(q2 + 2*q3) + 8*D3*L1^2*L2*L3*m3^2*q3_p*cos(2*q2 + q3) + 4*I3_zz*L1^3*L2*m1*m2*q1_p^2*sin(q2) + 8*I3_zz*L1^3*L2*m1*m3*q1_p^2*sin(q2) + 24*I3_zz*L1*L2^3*m2*m3*q1_p^2*sin(q2) + 48*I3_zz*L1^3*L2*m2*m3*q1_p^2*sin(q2) + 24*I3_zz*L1*L2^3*m2*m3*q2_p^2*sin(q2) + 8*I3_zz*L1*L2^3*m2^2*q1_p*q2_p*sin(q2) + 64*I3_zz*L1*L2^3*m3^2*q1_p*q2_p*sin(q2) - 8*I1_zz*L2*L3^3*m3^2*q1_p*q2_p*sin(q3) - 8*I1_zz*L2*L3^3*m3^2*q1_p*q3_p*sin(q3) - 8*I1_zz*L2*L3^3*m3^2*q2_p*q3_p*sin(q3) - 16*D1*I3_zz*L1*L2*m2*q1_p*cos(q2) - 32*D1*I3_zz*L1*L2*m3*q1_p*cos(q2) + 32*D2*I3_zz*L1*L2*m2*q2_p*cos(q2) + 64*D2*I3_zz*L1*L2*m3*q2_p*cos(q2) - 16*D3*I3_zz*L1*L2*m2*q3_p*cos(q2) - 32*D3*I3_zz*L1*L2*m3*q3_p*cos(q2) - 16*D3*I1_zz*L2*L3*m3*q3_p*cos(q3) + 8*I3_zz*L1*L2^2*L3*m3^2*q1_p^2*sin(q2 + q3) + 8*I3_zz*L1*L2^2*L3*m3^2*q2_p^2*sin(q2 + q3) + 8*I3_zz*L1*L2^2*L3*m3^2*q3_p^2*sin(q2 + q3) - 60*L1^2*L2*L3^2*g*m2*m3*cos(q1 - q2) + 25*L1*L2^2*L3^2*g*m2*m3*cos(q1 + 2*q2) - 10*L1*L2^2*L3^2*g*m2*m3*cos(q1 + 2*q3) + 4*I1_zz*L1*L2*L3^2*m3^2*q1_p^2*sin(q2) + 4*I2_zz*L1*L2*L3^2*m3^2*q1_p^2*sin(q2) + 4*I2_zz*L1*L2*L3^2*m3^2*q2_p^2*sin(q2) - 8*I3_zz*L1^2*L2*L3*m3^2*q1_p^2*sin(q3) - 8*I3_zz*L1^2*L2*L3*m3^2*q2_p^2*sin(q3) - 8*I3_zz*L1^2*L2*L3*m3^2*q3_p^2*sin(q3) + 16*I2_zz*I3_zz*L1*L3*m3*q1_p^2*sin(q2 + q3) + 16*I2_zz*I3_zz*L1*L3*m3*q2_p^2*sin(q2 + q3) + 16*I2_zz*I3_zz*L1*L3*m3*q3_p^2*sin(q2 + q3) - 4*I1_zz*L1*L2*L3^2*m3^2*q1_p^2*sin(q2 + 2*q3) + 4*I2_zz*L1*L2*L3^2*m3^2*q1_p^2*sin(q2 + 2*q3) + 8*I3_zz*L1*L2^2*L3*m3^2*q1_p^2*sin(q2 - q3) + 4*I2_zz*L1*L2*L3^2*m3^2*q2_p^2*sin(q2 + 2*q3) + 8*I3_zz*L1*L2^2*L3*m3^2*q2_p^2*sin(q2 - q3) + 8*I3_zz*L1^2*L2*L3*m3^2*q1_p^2*sin(2*q2 + q3) + 8*I3_zz*L1*L2^2*L3*m3^2*q3_p^2*sin(q2 - q3) + 8*I3_zz*L1^2*L2*L3*m3^2*q2_p^2*sin(2*q2 + q3) + 8*I3_zz*L1^2*L2*L3*m3^2*q3_p^2*sin(2*q2 + q3) + 16*I1_zz*I3_zz*L1*L2*m2*q1_p^2*sin(q2) + 32*I1_zz*I3_zz*L1*L2*m3*q1_p^2*sin(q2) + 16*I2_zz*I3_zz*L1*L2*m2*q1_p^2*sin(q2) + 16*I2_zz*I3_zz*L1*L2*m2*q2_p^2*sin(q2) + 32*I2_zz*I3_zz*L1*L2*m3*q1_p^2*sin(q2) + 32*I2_zz*I3_zz*L1*L2*m3*q2_p^2*sin(q2) - 16*I1_zz*I3_zz*L2*L3*m3*q1_p^2*sin(q3) - 16*I1_zz*I3_zz*L2*L3*m3*q2_p^2*sin(q3) - 16*I1_zz*I3_zz*L2*L3*m3*q3_p^2*sin(q3) - L1^2*L2^2*L3^2*m1*m3^2*q1_p^2*sin(2*q3) + 4*L1^2*L2^2*L3^2*m2*m3^2*q1_p^2*sin(2*q2) + 2*L1^2*L2^2*L3^2*m2^2*m3*q1_p^2*sin(2*q2) - L1^2*L2^2*L3^2*m1*m3^2*q2_p^2*sin(2*q3) - 2*L1^2*L2^2*L3^2*m2*m3^2*q1_p^2*sin(2*q3) + 2*L1^2*L2^2*L3^2*m2*m3^2*q2_p^2*sin(2*q2) + L1^2*L2^2*L3^2*m2^2*m3*q2_p^2*sin(2*q2) - 2*L1^2*L2^2*L3^2*m2*m3^2*q2_p^2*sin(2*q3) - 10*L1^2*L2*L3^2*g*m1*m3*cos(q1 + q2 + 2*q3) - 30*L1^2*L2*L3^2*g*m2*m3*cos(q1 + q2 + 2*q3) + 4*L1*L2*L3^2*m2*m3*tau1*cos(q2) - 8*L1*L2*L3^2*m2*m3*tau2*cos(q2) + 4*L1*L2*L3^2*m2*m3*tau3*cos(q2) + 4*L1^2*L2*L3*m1*m3*tau3*cos(q3) + 12*L1^2*L2*L3*m2*m3*tau3*cos(q3) + 8*D3*L1*L2^2*L3*m3^2*q3_p*cos(q2 + q3) - L1^2*L2^2*L3^2*m2*m3^2*q1_p^2*sin(2*q2 + 2*q3) + 25*L1^2*L2*L3^2*g*m1*m3*cos(q1 + q2) + 40*L1^2*L2*L3^2*g*m2*m3*cos(q1 + q2) + 32*I3_zz*L1^2*L2^2*m2*m3*q1_p^2*sin(2*q2) + 16*I3_zz*L1^2*L2^2*m2*m3*q2_p^2*sin(2*q2) + L1^3*L2*L3^2*m1*m3^2*q1_p^2*sin(q2) + 3*L1*L2^3*L3^2*m2*m3^2*q1_p^2*sin(q2) + L1*L2^3*L3^2*m2^2*m3*q1_p^2*sin(q2) - L1^2*L2*L3^3*m1*m3^2*q1_p^2*sin(q3) + 6*L1^3*L2*L3^2*m2*m3^2*q1_p^2*sin(q2) + 4*L1^3*L2*L3^2*m2^2*m3*q1_p^2*sin(q2) + 3*L1*L2^3*L3^2*m2*m3^2*q2_p^2*sin(q2) + L1*L2^3*L3^2*m2^2*m3*q2_p^2*sin(q2) - L1^2*L2*L3^3*m1*m3^2*q2_p^2*sin(q3) - 3*L1^2*L2*L3^3*m2*m3^2*q1_p^2*sin(q3) - L1^2*L2*L3^3*m1*m3^2*q3_p^2*sin(q3) - 3*L1^2*L2*L3^3*m2*m3^2*q2_p^2*sin(q3) - 3*L1^2*L2*L3^3*m2*m3^2*q3_p^2*sin(q3) + 8*I3_zz*L1^2*L2^2*m2^2*q1_p*q2_p*sin(2*q2) + 32*I3_zz*L1^2*L2^2*m3^2*q1_p*q2_p*sin(2*q2) - 8*I1_zz*L2^2*L3^2*m3^2*q1_p*q2_p*sin(2*q3) + 4*L1*L2^2*L3*m2*m3*tau3*cos(q2 - q3) - 4*L1^2*L2*L3*m2*m3*tau3*cos(2*q2 + q3) - 4*D1*L1*L2*L3^2*m3^2*q1_p*cos(q2) + 8*D2*L1*L2*L3^2*m3^2*q2_p*cos(q2) - 4*D3*L1*L2*L3^2*m3^2*q3_p*cos(q2) - 8*D3*L1^2*L2*L3*m3^2*q3_p*cos(q3) + 6*L1*L2^3*L3^2*m2*m3^2*q1_p*q2_p*sin(q2) + 2*L1*L2^3*L3^2*m2^2*m3*q1_p*q2_p*sin(q2) - 2*L1^2*L2*L3^3*m1*m3^2*q1_p*q2_p*sin(q3) - 2*L1^2*L2*L3^3*m1*m3^2*q1_p*q3_p*sin(q3) - 6*L1^2*L2*L3^3*m2*m3^2*q1_p*q2_p*sin(q3) - 2*L1^2*L2*L3^3*m1*m3^2*q2_p*q3_p*sin(q3) - 6*L1^2*L2*L3^3*m2*m3^2*q1_p*q3_p*sin(q3) - 6*L1^2*L2*L3^3*m2*m3^2*q2_p*q3_p*sin(q3) - 4*D1*L1*L2*L3^2*m2*m3*q1_p*cos(q2) + 8*D2*L1*L2*L3^2*m2*m3*q2_p*cos(q2) - 4*D3*L1*L2*L3^2*m2*m3*q3_p*cos(q2) - 4*D3*L1^2*L2*L3*m1*m3*q3_p*cos(q3) - 12*D3*L1^2*L2*L3*m2*m3*q3_p*cos(q3) + 2*L1*L2^2*L3^3*m2*m3^2*q1_p*q2_p*sin(q2 - q3) + 2*L1*L2^2*L3^3*m2*m3^2*q1_p*q3_p*sin(q2 - q3) - 2*L1*L2^3*L3^2*m2*m3^2*q1_p*q2_p*sin(q2 + 2*q3) + 2*L1^2*L2*L3^3*m2*m3^2*q1_p*q2_p*sin(2*q2 + q3) + 2*L1*L2^2*L3^3*m2*m3^2*q2_p*q3_p*sin(q2 - q3) + 2*L1^2*L2*L3^3*m2*m3^2*q1_p*q3_p*sin(2*q2 + q3) + 2*L1^2*L2*L3^3*m2*m3^2*q2_p*q3_p*sin(2*q2 + q3) - 4*D3*L1*L2^2*L3*m2*m3*q3_p*cos(q2 - q3) + 4*D3*L1^2*L2*L3*m2*m3*q3_p*cos(2*q2 + q3) + 48*I3_zz*L1*L2^3*m2*m3*q1_p*q2_p*sin(q2) + 16*I3_zz*L1*L2^2*L3*m3^2*q1_p*q2_p*sin(q2 + q3) + 16*I3_zz*L1*L2^2*L3*m3^2*q1_p*q3_p*sin(q2 + q3) + 16*I3_zz*L1*L2^2*L3*m3^2*q2_p*q3_p*sin(q2 + q3) + 4*I1_zz*L1*L2*L3^2*m2*m3*q1_p^2*sin(q2) + 4*I2_zz*L1*L2*L3^2*m2*m3*q1_p^2*sin(q2) + 4*I2_zz*L1*L2*L3^2*m2*m3*q2_p^2*sin(q2) - 4*I3_zz*L1^2*L2*L3*m1*m3*q1_p^2*sin(q3) - 4*I3_zz*L1^2*L2*L3*m1*m3*q2_p^2*sin(q3) - 12*I3_zz*L1^2*L2*L3*m2*m3*q1_p^2*sin(q3) - 4*I3_zz*L1^2*L2*L3*m1*m3*q3_p^2*sin(q3) - 12*I3_zz*L1^2*L2*L3*m2*m3*q2_p^2*sin(q3) - 12*I3_zz*L1^2*L2*L3*m2*m3*q3_p^2*sin(q3) + 8*I2_zz*L1*L2*L3^2*m3^2*q1_p*q2_p*sin(q2) - 16*I3_zz*L1^2*L2*L3*m3^2*q1_p*q2_p*sin(q3) - 16*I3_zz*L1^2*L2*L3*m3^2*q1_p*q3_p*sin(q3) - 16*I3_zz*L1^2*L2*L3*m3^2*q2_p*q3_p*sin(q3) + 32*I2_zz*I3_zz*L1*L3*m3*q1_p*q2_p*sin(q2 + q3) + 32*I2_zz*I3_zz*L1*L3*m3*q1_p*q3_p*sin(q2 + q3) + 32*I2_zz*I3_zz*L1*L3*m3*q2_p*q3_p*sin(q2 + q3) + 4*I3_zz*L1*L2^2*L3*m2*m3*q1_p^2*sin(q2 - q3) + 4*I3_zz*L1*L2^2*L3*m2*m3*q2_p^2*sin(q2 - q3) + 4*I3_zz*L1^2*L2*L3*m2*m3*q1_p^2*sin(2*q2 + q3) + 4*I3_zz*L1*L2^2*L3*m2*m3*q3_p^2*sin(q2 - q3) + 4*I3_zz*L1^2*L2*L3*m2*m3*q2_p^2*sin(2*q2 + q3) + 4*I3_zz*L1^2*L2*L3*m2*m3*q3_p^2*sin(2*q2 + q3) + 8*I2_zz*L1*L2*L3^2*m3^2*q1_p*q2_p*sin(q2 + 2*q3) + 16*I3_zz*L1*L2^2*L3*m3^2*q1_p*q2_p*sin(q2 - q3) + 16*I3_zz*L1*L2^2*L3*m3^2*q1_p*q3_p*sin(q2 - q3) + 16*I3_zz*L1^2*L2*L3*m3^2*q1_p*q2_p*sin(2*q2 + q3) + 16*I3_zz*L1*L2^2*L3*m3^2*q2_p*q3_p*sin(q2 - q3) + 16*I3_zz*L1^2*L2*L3*m3^2*q1_p*q3_p*sin(2*q2 + q3) + 16*I3_zz*L1^2*L2*L3*m3^2*q2_p*q3_p*sin(2*q2 + q3) + 32*I2_zz*I3_zz*L1*L2*m2*q1_p*q2_p*sin(q2) + 64*I2_zz*I3_zz*L1*L2*m3*q1_p*q2_p*sin(q2) - 32*I1_zz*I3_zz*L2*L3*m3*q1_p*q2_p*sin(q3) - 32*I1_zz*I3_zz*L2*L3*m3*q1_p*q3_p*sin(q3) - 32*I1_zz*I3_zz*L2*L3*m3*q2_p*q3_p*sin(q3) - 2*L1^2*L2^2*L3^2*m1*m3^2*q1_p*q2_p*sin(2*q3) + 4*L1^2*L2^2*L3^2*m2*m3^2*q1_p*q2_p*sin(2*q2) + 2*L1^2*L2^2*L3^2*m2^2*m3*q1_p*q2_p*sin(2*q2) - 4*L1^2*L2^2*L3^2*m2*m3^2*q1_p*q2_p*sin(2*q3) + L1^3*L2*L3^2*m1*m2*m3*q1_p^2*sin(q2) + 32*I3_zz*L1^2*L2^2*m2*m3*q1_p*q2_p*sin(2*q2) + 8*I2_zz*L1*L2*L3^2*m2*m3*q1_p*q2_p*sin(q2) - 8*I3_zz*L1^2*L2*L3*m1*m3*q1_p*q2_p*sin(q3) - 8*I3_zz*L1^2*L2*L3*m1*m3*q1_p*q3_p*sin(q3) - 24*I3_zz*L1^2*L2*L3*m2*m3*q1_p*q2_p*sin(q3) - 8*I3_zz*L1^2*L2*L3*m1*m3*q2_p*q3_p*sin(q3) - 24*I3_zz*L1^2*L2*L3*m2*m3*q1_p*q3_p*sin(q3) - 24*I3_zz*L1^2*L2*L3*m2*m3*q2_p*q3_p*sin(q3) + 8*I3_zz*L1*L2^2*L3*m2*m3*q1_p*q2_p*sin(q2 - q3) + 8*I3_zz*L1*L2^2*L3*m2*m3*q1_p*q3_p*sin(q2 - q3) + 8*I3_zz*L1^2*L2*L3*m2*m3*q1_p*q2_p*sin(2*q2 + q3) + 8*I3_zz*L1*L2^2*L3*m2*m3*q2_p*q3_p*sin(q2 - q3) + 8*I3_zz*L1^2*L2*L3*m2*m3*q1_p*q3_p*sin(2*q2 + q3) + 8*I3_zz*L1^2*L2*L3*m2*m3*q2_p*q3_p*sin(2*q2 + q3)))/(64*I1_zz*I2_zz*I3_zz + 16*I2_zz*I3_zz*L1^2*m1 + 16*I1_zz*I3_zz*L2^2*m2 + 64*I2_zz*I3_zz*L1^2*m2 + 16*I1_zz*I2_zz*L3^2*m3 + 64*I1_zz*I3_zz*L2^2*m3 + 64*I2_zz*I3_zz*L1^2*m3 + 8*I3_zz*L1^2*L2^2*m2^2 + 8*I1_zz*L2^2*L3^2*m3^2 + 8*I2_zz*L1^2*L3^2*m3^2 + 32*I3_zz*L1^2*L2^2*m3^2 - 8*I2_zz*L1^2*L3^2*m3^2*cos(2*q2 + 2*q3) + 2*L1^2*L2^2*L3^2*m1*m3^2 + 6*L1^2*L2^2*L3^2*m2*m3^2 + 2*L1^2*L2^2*L3^2*m2^2*m3 + 4*I3_zz*L1^2*L2^2*m1*m2 + 4*I2_zz*L1^2*L3^2*m1*m3 + 16*I3_zz*L1^2*L2^2*m1*m3 + 4*I1_zz*L2^2*L3^2*m2*m3 + 16*I2_zz*L1^2*L3^2*m2*m3 + 48*I3_zz*L1^2*L2^2*m2*m3 - 8*I3_zz*L1^2*L2^2*m2^2*cos(2*q2) - 32*I3_zz*L1^2*L2^2*m3^2*cos(2*q2) - 8*I1_zz*L2^2*L3^2*m3^2*cos(2*q3) - 32*I3_zz*L1^2*L2^2*m2*m3*cos(2*q2) + L1^2*L2^2*L3^2*m1*m2*m3 - 2*L1^2*L2^2*L3^2*m1*m3^2*cos(2*q3) - 4*L1^2*L2^2*L3^2*m2*m3^2*cos(2*q2) - 2*L1^2*L2^2*L3^2*m2^2*m3*cos(2*q2) - 4*L1^2*L2^2*L3^2*m2*m3^2*cos(2*q3) + 2*L1^2*L2^2*L3^2*m2*m3^2*cos(2*q2 + 2*q3));
    q3_pp = -(2*(32*I1_zz*I3_zz*tau2 - 32*I1_zz*I2_zz*tau3 - 32*I1_zz*I3_zz*tau3 - 8*I2_zz*L1^2*m1*tau3 + 8*I3_zz*L1^2*m1*tau2 - 8*I1_zz*L2^2*m2*tau3 - 32*I2_zz*L1^2*m2*tau3 - 8*I3_zz*L1^2*m1*tau3 + 32*I3_zz*L1^2*m2*tau2 - 32*I1_zz*L2^2*m3*tau3 + 8*I1_zz*L3^2*m3*tau2 - 32*I2_zz*L1^2*m3*tau3 - 32*I3_zz*L1^2*m2*tau3 + 32*I3_zz*L1^2*m3*tau2 - 8*I1_zz*L3^2*m3*tau3 - 32*I3_zz*L1^2*m3*tau3 - 32*D2*I1_zz*I3_zz*q2_p + 32*D3*I1_zz*I2_zz*q3_p + 32*D3*I1_zz*I3_zz*q3_p - 4*L1^2*L2^2*m2^2*tau3 - 16*L1^2*L2^2*m3^2*tau3 + 4*L1^2*L3^2*m3^2*tau2 - 4*L1^2*L3^2*m3^2*tau3 - 2*L1^2*L2^2*m1*m2*tau3 - 8*L1^2*L2^2*m1*m3*tau3 + 2*L1^2*L3^2*m1*m3*tau2 - 24*L1^2*L2^2*m2*m3*tau3 - 2*L1^2*L3^2*m1*m3*tau3 + 8*L1^2*L3^2*m2*m3*tau2 - 8*L1^2*L3^2*m2*m3*tau3 + 4*L1^2*L2^2*m2^2*tau3*cos(2*q2) + 16*L1^2*L2^2*m3^2*tau3*cos(2*q2) - 4*D2*L1^2*L3^2*m3^2*q2_p + 4*D3*L1^2*L2^2*m2^2*q3_p + 16*D3*L1^2*L2^2*m3^2*q3_p + 4*D3*L1^2*L3^2*m3^2*q3_p - 560*I1_zz*I3_zz*L2*g*cos(q1 + q2) - 4*L1^2*L3^2*m3^2*tau2*cos(2*q2 + 2*q3) + 4*L1^2*L3^2*m3^2*tau3*cos(2*q2 + 2*q3) - 8*D2*I3_zz*L1^2*m1*q2_p - 32*D2*I3_zz*L1^2*m2*q2_p + 8*D3*I2_zz*L1^2*m1*q3_p - 8*D2*I1_zz*L3^2*m3*q2_p - 32*D2*I3_zz*L1^2*m3*q2_p + 8*D3*I1_zz*L2^2*m2*q3_p + 32*D3*I2_zz*L1^2*m2*q3_p + 8*D3*I3_zz*L1^2*m1*q3_p + 32*D3*I1_zz*L2^2*m3*q3_p + 32*D3*I2_zz*L1^2*m3*q3_p + 32*D3*I3_zz*L1^2*m2*q3_p + 8*D3*I1_zz*L3^2*m3*q3_p + 32*D3*I3_zz*L1^2*m3*q3_p + 160*I1_zz*I2_zz*L3*g*cos(q1 + q2 + q3) - 70*L1^2*L2^2*L3*g*m3^2*cos(q1 - q2 - q3) - 35*L1^2*L2*L3^2*g*m3^2*cos(q1 - q2 - 2*q3) + 15*L1^2*L2*L3^2*g*m3^2*cos(q1 + 3*q2 + 2*q3) + 4*I2_zz*L1^2*L3^2*m3^2*q1_p^2*sin(2*q2 + 2*q3) + 4*I2_zz*L1^2*L3^2*m3^2*q2_p^2*sin(2*q2 + 2*q3) + 4*I2_zz*L1^2*L3^2*m3^2*q3_p^2*sin(2*q2 + 2*q3) - 140*I3_zz*L1^2*L2*g*m1*cos(q1 + q2) - 280*I3_zz*L1^2*L2*g*m2*cos(q1 + q2) - 100*I1_zz*L2*L3^2*g*m3*cos(q1 + q2) - 16*I3_zz*L1^3*L2*m2^2*q1_p^2*sin(q2) - 32*I3_zz*L1^3*L2*m3^2*q1_p^2*sin(q2) + 4*I1_zz*L2*L3^3*m3^2*q1_p^2*sin(q3) + 16*I1_zz*L2^3*L3*m3^2*q1_p^2*sin(q3) + 4*I1_zz*L2*L3^3*m3^2*q2_p^2*sin(q3) + 16*I1_zz*L2^3*L3*m3^2*q2_p^2*sin(q3) + 4*I1_zz*L2*L3^3*m3^2*q3_p^2*sin(q3) + 16*L1^2*L2^2*m2*m3*tau3*cos(2*q2) + 50*L1^2*L2*L3^2*g*m3^2*cos(q1 - q2) - 2*D2*L1^2*L3^2*m1*m3*q2_p + 2*D3*L1^2*L2^2*m1*m2*q3_p - 8*D2*L1^2*L3^2*m2*m3*q2_p + 8*D3*L1^2*L2^2*m1*m3*q3_p + 24*D3*L1^2*L2^2*m2*m3*q3_p + 2*D3*L1^2*L3^2*m1*m3*q3_p + 8*D3*L1^2*L3^2*m2*m3*q3_p - 280*I2_zz*L1^2*L3*g*m3*cos(q1 - q2 - q3) + 20*L1^2*L2^2*L3*g*m2^2*cos(q1 + q2 + q3) - 130*L1^2*L2^2*L3*g*m3^2*cos(q1 + q2 + q3) - 4*D3*L1^2*L2^2*m2^2*q3_p*cos(2*q2) - 16*D3*L1^2*L2^2*m3^2*q3_p*cos(2*q2) + 280*I3_zz*L1^2*L2*g*m2*cos(q1 - q2) + 560*I3_zz*L1^2*L2*g*m3*cos(q1 - q2) + 8*L1*L2^2*L3*m3^2*tau1*cos(q2 + q3) - 8*L1*L2^2*L3*m3^2*tau2*cos(q2 + q3) + 40*I2_zz*L1^2*L3*g*m1*cos(q1 + q2 + q3) + 40*I1_zz*L2^2*L3*g*m2*cos(q1 + q2 + q3) + 160*I2_zz*L1^2*L3*g*m2*cos(q1 + q2 + q3) + 20*I1_zz*L2^2*L3*g*m3*cos(q1 + q2 + q3) - 120*I2_zz*L1^2*L3*g*m3*cos(q1 + q2 + q3) + 4*D2*L1^2*L3^2*m3^2*q2_p*cos(2*q2 + 2*q3) - 4*D3*L1^2*L3^2*m3^2*q3_p*cos(2*q2 + 2*q3) - 10*L1^2*L2^2*L3*g*m2^2*cos(q1 - q2 + q3) + 70*L1^2*L2^2*L3*g*m3^2*cos(q1 + q2 - q3) + 100*L1^2*L2^2*L3*g*m3^2*cos(q1 - q2 + q3) - 50*L1^2*L2*L3^2*g*m3^2*cos(q1 + q2 + 2*q3) - 10*L1^2*L2^2*L3*g*m2^2*cos(q1 + 3*q2 + q3) + 30*L1^2*L2^2*L3*g*m3^2*cos(q1 + 3*q2 + q3) - 4*L1*L2*L3^2*m3^2*tau1*cos(q2) + 4*L1*L2*L3^2*m3^2*tau2*cos(q2) + 8*L1^2*L2*L3*m3^2*tau2*cos(q3) - 16*L1^2*L2*L3*m3^2*tau3*cos(q3) + 16*I2_zz*L1*L3*m3*tau1*cos(q2 + q3) - 16*I2_zz*L1*L3*m3*tau2*cos(q2 + q3) + 20*L1^2*L2*L3^2*g*m3^2*cos(q1 + q2) - 4*I3_zz*L1^2*L2^2*m2^2*q1_p^2*sin(2*q2) - 4*I3_zz*L1^2*L2^2*m2^2*q2_p^2*sin(2*q2) - 16*I3_zz*L1^2*L2^2*m3^2*q1_p^2*sin(2*q2) + 8*I1_zz*L2^2*L3^2*m3^2*q1_p^2*sin(2*q3) - 16*I3_zz*L1^2*L2^2*m3^2*q2_p^2*sin(2*q2) + 8*I1_zz*L2^2*L3^2*m3^2*q2_p^2*sin(2*q3) + 4*I1_zz*L2^2*L3^2*m3^2*q3_p^2*sin(2*q3) - 8*L1*L2^2*L3*m3^2*tau1*cos(q2 - q3) + 4*L1*L2*L3^2*m3^2*tau1*cos(q2 + 2*q3) + 8*L1*L2^2*L3*m3^2*tau2*cos(q2 - q3) - 4*L1*L2*L3^2*m3^2*tau2*cos(q2 + 2*q3) - 8*L1^2*L2*L3*m3^2*tau2*cos(2*q2 + q3) + 16*L1^2*L2*L3*m3^2*tau3*cos(2*q2 + q3) - 140*I1_zz*L2^2*L3*g*m3*cos(q1 + q2 - q3) + 40*I1_zz*L2*L3^2*g*m3*cos(q1 + q2 + 2*q3) + 16*I2_zz*L1^3*L3*m3^2*q1_p^2*sin(q2 + q3) - 16*I3_zz*L1*L2*m2*tau1*cos(q2) + 16*I3_zz*L1*L2*m2*tau2*cos(q2) - 32*I3_zz*L1*L2*m3*tau1*cos(q2) + 32*I3_zz*L1*L2*m3*tau2*cos(q2) + 16*I1_zz*L2*L3*m3*tau2*cos(q3) - 32*I1_zz*L2*L3*m3*tau3*cos(q3) - 16*D1*I2_zz*L1*L3*m3*q1_p*cos(q2 + q3) + 16*D2*I2_zz*L1*L3*m3*q2_p*cos(q2 + q3) + 35*L1^2*L2^2*L3*g*m2*m3*cos(q1 - q2 - q3) - 10*L1^2*L2*L3^2*g*m2*m3*cos(q1 + 3*q2 + 2*q3) - 2*L1^3*L2^2*L3*m1*m3^2*q1_p^2*sin(q2 - q3) + L1^3*L2*L3^2*m1*m3^2*q1_p^2*sin(q2 + 2*q3) - 4*L1^3*L2^2*L3*m2*m3^2*q1_p^2*sin(q2 - q3) - 2*L1^3*L2^2*L3*m2^2*m3*q1_p^2*sin(q2 - q3) - L1^2*L2*L3^3*m2*m3^2*q1_p^2*sin(2*q2 + q3) - 2*L1^2*L2^3*L3*m2*m3^2*q1_p^2*sin(2*q2 + q3) - L1^2*L2^3*L3*m2^2*m3*q1_p^2*sin(2*q2 + q3) + 2*L1^3*L2*L3^2*m2*m3^2*q1_p^2*sin(q2 + 2*q3) - L1^2*L2*L3^3*m2*m3^2*q2_p^2*sin(2*q2 + q3) - 2*L1^2*L2^3*L3*m2*m3^2*q2_p^2*sin(2*q2 + q3) - L1^2*L2^3*L3*m2^2*m3*q2_p^2*sin(2*q2 + q3) - L1^2*L2*L3^3*m2*m3^2*q3_p^2*sin(2*q2 + q3) + 8*I2_zz*L1^2*L3^2*m3^2*q1_p*q2_p*sin(2*q2 + 2*q3) + 8*I2_zz*L1^2*L3^2*m3^2*q1_p*q3_p*sin(2*q2 + 2*q3) + 8*I2_zz*L1^2*L3^2*m3^2*q2_p*q3_p*sin(2*q2 + 2*q3) + 8*D1*L1*L2^2*L3*m3^2*q1_p*cos(q2 - q3) - 4*D1*L1*L2*L3^2*m3^2*q1_p*cos(q2 + 2*q3) - 8*D2*L1*L2^2*L3*m3^2*q2_p*cos(q2 - q3) + 4*D2*L1*L2*L3^2*m3^2*q2_p*cos(q2 + 2*q3) + 8*D2*L1^2*L2*L3*m3^2*q2_p*cos(2*q2 + q3) - 16*D3*L1^2*L2*L3*m3^2*q3_p*cos(2*q2 + q3) - 4*I3_zz*L1^3*L2*m1*m2*q1_p^2*sin(q2) - 8*I3_zz*L1^3*L2*m1*m3*q1_p^2*sin(q2) - 48*I3_zz*L1^3*L2*m2*m3*q1_p^2*sin(q2) + 4*I1_zz*L2^3*L3*m2*m3*q1_p^2*sin(q3) + 4*I1_zz*L2^3*L3*m2*m3*q2_p^2*sin(q3) + 8*I1_zz*L2*L3^3*m3^2*q1_p*q2_p*sin(q3) + 32*I1_zz*L2^3*L3*m3^2*q1_p*q2_p*sin(q3) + 8*I1_zz*L2*L3^3*m3^2*q1_p*q3_p*sin(q3) + 8*I1_zz*L2*L3^3*m3^2*q2_p*q3_p*sin(q3) + 16*D1*I3_zz*L1*L2*m2*q1_p*cos(q2) + 32*D1*I3_zz*L1*L2*m3*q1_p*cos(q2) - 16*D2*I3_zz*L1*L2*m2*q2_p*cos(q2) - 32*D2*I3_zz*L1*L2*m3*q2_p*cos(q2) - 16*D2*I1_zz*L2*L3*m3*q2_p*cos(q3) + 32*D3*I1_zz*L2*L3*m3*q3_p*cos(q3) + 8*I1_zz*L1*L2^2*L3*m3^2*q1_p^2*sin(q2 + q3) + 60*L1^2*L2*L3^2*g*m2*m3*cos(q1 - q2) + 10*L1^2*L2^2*L3*g*m1*m2*cos(q1 + q2 + q3) + 5*L1^2*L2^2*L3*g*m1*m3*cos(q1 + q2 + q3) + 15*L1^2*L2^2*L3*g*m2*m3*cos(q1 + q2 + q3) - 4*I1_zz*L1*L2*L3^2*m3^2*q1_p^2*sin(q2) + 8*I2_zz*L1^2*L2*L3*m3^2*q1_p^2*sin(q3) + 8*I2_zz*L1^2*L2*L3*m3^2*q2_p^2*sin(q3) + 8*I3_zz*L1^2*L2*L3*m3^2*q1_p^2*sin(q3) + 8*I3_zz*L1^2*L2*L3*m3^2*q2_p^2*sin(q3) + 8*I3_zz*L1^2*L2*L3*m3^2*q3_p^2*sin(q3) - 16*D3*L1^2*L2^2*m2*m3*q3_p*cos(2*q2) + 16*I1_zz*I2_zz*L1*L3*m3*q1_p^2*sin(q2 + q3) - 8*I1_zz*L1*L2^2*L3*m3^2*q1_p^2*sin(q2 - q3) + 4*I1_zz*L1*L2*L3^2*m3^2*q1_p^2*sin(q2 + 2*q3) + 8*I2_zz*L1^2*L2*L3*m3^2*q1_p^2*sin(2*q2 + q3) + 8*I2_zz*L1^2*L2*L3*m3^2*q2_p^2*sin(2*q2 + q3) - 8*I3_zz*L1^2*L2*L3*m3^2*q1_p^2*sin(2*q2 + q3) - 8*I3_zz*L1^2*L2*L3*m3^2*q2_p^2*sin(2*q2 + q3) - 8*I3_zz*L1^2*L2*L3*m3^2*q3_p^2*sin(2*q2 + q3) - 16*I1_zz*I3_zz*L1*L2*m2*q1_p^2*sin(q2) - 32*I1_zz*I3_zz*L1*L2*m3*q1_p^2*sin(q2) + 16*I1_zz*I2_zz*L2*L3*m3*q1_p^2*sin(q3) + 16*I1_zz*I2_zz*L2*L3*m3*q2_p^2*sin(q3) + 16*I1_zz*I3_zz*L2*L3*m3*q1_p^2*sin(q3) + 16*I1_zz*I3_zz*L2*L3*m3*q2_p^2*sin(q3) + 16*I1_zz*I3_zz*L2*L3*m3*q3_p^2*sin(q3) + 2*L1^2*L2^2*L3^2*m1*m3^2*q1_p^2*sin(2*q3) - 2*L1^2*L2^2*L3^2*m2*m3^2*q1_p^2*sin(2*q2) - L1^2*L2^2*L3^2*m2^2*m3*q1_p^2*sin(2*q2) + 2*L1^2*L2^2*L3^2*m1*m3^2*q2_p^2*sin(2*q3) + 4*L1^2*L2^2*L3^2*m2*m3^2*q1_p^2*sin(2*q3) - 2*L1^2*L2^2*L3^2*m2*m3^2*q2_p^2*sin(2*q2) - L1^2*L2^2*L3^2*m2^2*m3*q2_p^2*sin(2*q2) + L1^2*L2^2*L3^2*m1*m3^2*q3_p^2*sin(2*q3) + 4*L1^2*L2^2*L3^2*m2*m3^2*q2_p^2*sin(2*q3) + 2*L1^2*L2^2*L3^2*m2*m3^2*q3_p^2*sin(2*q3) - 35*L1^2*L2^2*L3*g*m1*m3*cos(q1 + q2 - q3) + 10*L1^2*L2*L3^2*g*m1*m3*cos(q1 + q2 + 2*q3) - 35*L1^2*L2^2*L3*g*m2*m3*cos(q1 + q2 - q3) + 30*L1^2*L2^2*L3*g*m2*m3*cos(q1 - q2 + q3) + 30*L1^2*L2*L3^2*g*m2*m3*cos(q1 + q2 + 2*q3) - 5*L1^2*L2^2*L3*g*m2*m3*cos(q1 + 3*q2 + q3) + 2*L1^3*L2^2*L3*m1*m3^2*q1_p^2*sin(q2 + q3) - 2*L1^3*L2^2*L3*m2^2*m3*q1_p^2*sin(q2 + q3) - 4*L1*L2*L3^2*m2*m3*tau1*cos(q2) + 4*L1*L2*L3^2*m2*m3*tau2*cos(q2) + 4*L1^2*L2*L3*m1*m3*tau2*cos(q3) - 8*L1^2*L2*L3*m1*m3*tau3*cos(q3) + 12*L1^2*L2*L3*m2*m3*tau2*cos(q3) - 24*L1^2*L2*L3*m2*m3*tau3*cos(q3) - 8*D1*L1*L2^2*L3*m3^2*q1_p*cos(q2 + q3) + 8*D2*L1*L2^2*L3*m3^2*q2_p*cos(q2 + q3) - L1^2*L2^2*L3^2*m2*m3^2*q1_p^2*sin(2*q2 + 2*q3) - L1^2*L2^2*L3^2*m2*m3^2*q2_p^2*sin(2*q2 + 2*q3) - L1^2*L2^2*L3^2*m2*m3^2*q3_p^2*sin(2*q2 + 2*q3) - 25*L1^2*L2*L3^2*g*m1*m3*cos(q1 + q2) - 40*L1^2*L2*L3^2*g*m2*m3*cos(q1 + q2) - 16*I3_zz*L1^2*L2^2*m2*m3*q1_p^2*sin(2*q2) - 16*I3_zz*L1^2*L2^2*m2*m3*q2_p^2*sin(2*q2) - L1^3*L2*L3^2*m1*m3^2*q1_p^2*sin(q2) + L1^2*L2*L3^3*m1*m3^2*q1_p^2*sin(q3) + 4*L1^2*L2^3*L3*m1*m3^2*q1_p^2*sin(q3) - 6*L1^3*L2*L3^2*m2*m3^2*q1_p^2*sin(q2) - 4*L1^3*L2*L3^2*m2^2*m3*q1_p^2*sin(q2) + L1^2*L2*L3^3*m1*m3^2*q2_p^2*sin(q3) + 3*L1^2*L2*L3^3*m2*m3^2*q1_p^2*sin(q3) + 4*L1^2*L2^3*L3*m1*m3^2*q2_p^2*sin(q3) + 6*L1^2*L2^3*L3*m2*m3^2*q1_p^2*sin(q3) + L1^2*L2^3*L3*m2^2*m3*q1_p^2*sin(q3) + L1^2*L2*L3^3*m1*m3^2*q3_p^2*sin(q3) + 3*L1^2*L2*L3^3*m2*m3^2*q2_p^2*sin(q3) + 6*L1^2*L2^3*L3*m2*m3^2*q2_p^2*sin(q3) + L1^2*L2^3*L3*m2^2*m3*q2_p^2*sin(q3) + 3*L1^2*L2*L3^3*m2*m3^2*q3_p^2*sin(q3) - 8*I3_zz*L1^2*L2^2*m2^2*q1_p*q2_p*sin(2*q2) - 32*I3_zz*L1^2*L2^2*m3^2*q1_p*q2_p*sin(2*q2) + 16*I1_zz*L2^2*L3^2*m3^2*q1_p*q2_p*sin(2*q3) + 8*I1_zz*L2^2*L3^2*m3^2*q1_p*q3_p*sin(2*q3) + 8*I1_zz*L2^2*L3^2*m3^2*q2_p*q3_p*sin(2*q3) - 4*L1*L2^2*L3*m2*m3*tau1*cos(q2 - q3) + 4*L1*L2^2*L3*m2*m3*tau2*cos(q2 - q3) - 4*L1^2*L2*L3*m2*m3*tau2*cos(2*q2 + q3) + 8*L1^2*L2*L3*m2*m3*tau3*cos(2*q2 + q3) + 4*D1*L1*L2*L3^2*m3^2*q1_p*cos(q2) - 4*D2*L1*L2*L3^2*m3^2*q2_p*cos(q2) - 8*D2*L1^2*L2*L3*m3^2*q2_p*cos(q3) + 16*D3*L1^2*L2*L3*m3^2*q3_p*cos(q3) + 4*I2_zz*L1^3*L3*m1*m3*q1_p^2*sin(q2 + q3) + 16*I2_zz*L1^3*L3*m2*m3*q1_p^2*sin(q2 + q3) + 2*L1^2*L2*L3^3*m1*m3^2*q1_p*q2_p*sin(q3) + 8*L1^2*L2^3*L3*m1*m3^2*q1_p*q2_p*sin(q3) + 2*L1^2*L2*L3^3*m1*m3^2*q1_p*q3_p*sin(q3) + 6*L1^2*L2*L3^3*m2*m3^2*q1_p*q2_p*sin(q3) + 12*L1^2*L2^3*L3*m2*m3^2*q1_p*q2_p*sin(q3) + 2*L1^2*L2^3*L3*m2^2*m3*q1_p*q2_p*sin(q3) + 2*L1^2*L2*L3^3*m1*m3^2*q2_p*q3_p*sin(q3) + 6*L1^2*L2*L3^3*m2*m3^2*q1_p*q3_p*sin(q3) + 6*L1^2*L2*L3^3*m2*m3^2*q2_p*q3_p*sin(q3) + 4*D1*L1*L2*L3^2*m2*m3*q1_p*cos(q2) - 4*D2*L1*L2*L3^2*m2*m3*q2_p*cos(q2) - 4*D2*L1^2*L2*L3*m1*m3*q2_p*cos(q3) - 12*D2*L1^2*L2*L3*m2*m3*q2_p*cos(q3) + 8*D3*L1^2*L2*L3*m1*m3*q3_p*cos(q3) + 24*D3*L1^2*L2*L3*m2*m3*q3_p*cos(q3) - L1^3*L2^2*L3*m1*m2*m3*q1_p^2*sin(q2 - q3) - 2*L1^2*L2*L3^3*m2*m3^2*q1_p*q2_p*sin(2*q2 + q3) - 4*L1^2*L2^3*L3*m2*m3^2*q1_p*q2_p*sin(2*q2 + q3) - 2*L1^2*L2^3*L3*m2^2*m3*q1_p*q2_p*sin(2*q2 + q3) - 2*L1^2*L2*L3^3*m2*m3^2*q1_p*q3_p*sin(2*q2 + q3) - 2*L1^2*L2*L3^3*m2*m3^2*q2_p*q3_p*sin(2*q2 + q3) + 4*D1*L1*L2^2*L3*m2*m3*q1_p*cos(q2 - q3) - 4*D2*L1*L2^2*L3*m2*m3*q2_p*cos(q2 - q3) + 4*D2*L1^2*L2*L3*m2*m3*q2_p*cos(2*q2 + q3) - 8*D3*L1^2*L2*L3*m2*m3*q3_p*cos(2*q2 + q3) + 8*I1_zz*L2^3*L3*m2*m3*q1_p*q2_p*sin(q3) - 4*I1_zz*L1*L2*L3^2*m2*m3*q1_p^2*sin(q2) + 4*I2_zz*L1^2*L2*L3*m1*m3*q1_p^2*sin(q3) + 4*I2_zz*L1^2*L2*L3*m1*m3*q2_p^2*sin(q3) + 12*I2_zz*L1^2*L2*L3*m2*m3*q1_p^2*sin(q3) + 4*I3_zz*L1^2*L2*L3*m1*m3*q1_p^2*sin(q3) + 12*I2_zz*L1^2*L2*L3*m2*m3*q2_p^2*sin(q3) + 4*I3_zz*L1^2*L2*L3*m1*m3*q2_p^2*sin(q3) + 12*I3_zz*L1^2*L2*L3*m2*m3*q1_p^2*sin(q3) + 4*I3_zz*L1^2*L2*L3*m1*m3*q3_p^2*sin(q3) + 12*I3_zz*L1^2*L2*L3*m2*m3*q2_p^2*sin(q3) + 12*I3_zz*L1^2*L2*L3*m2*m3*q3_p^2*sin(q3) + 16*I2_zz*L1^2*L2*L3*m3^2*q1_p*q2_p*sin(q3) + 16*I3_zz*L1^2*L2*L3*m3^2*q1_p*q2_p*sin(q3) + 16*I3_zz*L1^2*L2*L3*m3^2*q1_p*q3_p*sin(q3) + 16*I3_zz*L1^2*L2*L3*m3^2*q2_p*q3_p*sin(q3) - 4*I1_zz*L1*L2^2*L3*m2*m3*q1_p^2*sin(q2 - q3) + 4*I2_zz*L1^2*L2*L3*m2*m3*q1_p^2*sin(2*q2 + q3) + 4*I2_zz*L1^2*L2*L3*m2*m3*q2_p^2*sin(2*q2 + q3) - 4*I3_zz*L1^2*L2*L3*m2*m3*q1_p^2*sin(2*q2 + q3) - 4*I3_zz*L1^2*L2*L3*m2*m3*q2_p^2*sin(2*q2 + q3) - 4*I3_zz*L1^2*L2*L3*m2*m3*q3_p^2*sin(2*q2 + q3) + 16*I2_zz*L1^2*L2*L3*m3^2*q1_p*q2_p*sin(2*q2 + q3) - 16*I3_zz*L1^2*L2*L3*m3^2*q1_p*q2_p*sin(2*q2 + q3) - 16*I3_zz*L1^2*L2*L3*m3^2*q1_p*q3_p*sin(2*q2 + q3) - 16*I3_zz*L1^2*L2*L3*m3^2*q2_p*q3_p*sin(2*q2 + q3) + 32*I1_zz*I2_zz*L2*L3*m3*q1_p*q2_p*sin(q3) + 32*I1_zz*I3_zz*L2*L3*m3*q1_p*q2_p*sin(q3) + 32*I1_zz*I3_zz*L2*L3*m3*q1_p*q3_p*sin(q3) + 32*I1_zz*I3_zz*L2*L3*m3*q2_p*q3_p*sin(q3) + 4*L1^2*L2^2*L3^2*m1*m3^2*q1_p*q2_p*sin(2*q3) - 4*L1^2*L2^2*L3^2*m2*m3^2*q1_p*q2_p*sin(2*q2) - 2*L1^2*L2^2*L3^2*m2^2*m3*q1_p*q2_p*sin(2*q2) + 2*L1^2*L2^2*L3^2*m1*m3^2*q1_p*q3_p*sin(2*q3) + 8*L1^2*L2^2*L3^2*m2*m3^2*q1_p*q2_p*sin(2*q3) + 2*L1^2*L2^2*L3^2*m1*m3^2*q2_p*q3_p*sin(2*q3) + 4*L1^2*L2^2*L3^2*m2*m3^2*q1_p*q3_p*sin(2*q3) + 4*L1^2*L2^2*L3^2*m2*m3^2*q2_p*q3_p*sin(2*q3) - 2*L1^2*L2^2*L3^2*m2*m3^2*q1_p*q2_p*sin(2*q2 + 2*q3) - 2*L1^2*L2^2*L3^2*m2*m3^2*q1_p*q3_p*sin(2*q2 + 2*q3) - 2*L1^2*L2^2*L3^2*m2*m3^2*q2_p*q3_p*sin(2*q2 + 2*q3) - L1^3*L2*L3^2*m1*m2*m3*q1_p^2*sin(q2) + L1^2*L2^3*L3*m1*m2*m3*q1_p^2*sin(q3) + L1^2*L2^3*L3*m1*m2*m3*q2_p^2*sin(q3) - 32*I3_zz*L1^2*L2^2*m2*m3*q1_p*q2_p*sin(2*q2) + 2*L1^2*L2^3*L3*m1*m2*m3*q1_p*q2_p*sin(q3) + 8*I2_zz*L1^2*L2*L3*m1*m3*q1_p*q2_p*sin(q3) + 24*I2_zz*L1^2*L2*L3*m2*m3*q1_p*q2_p*sin(q3) + 8*I3_zz*L1^2*L2*L3*m1*m3*q1_p*q2_p*sin(q3) + 8*I3_zz*L1^2*L2*L3*m1*m3*q1_p*q3_p*sin(q3) + 24*I3_zz*L1^2*L2*L3*m2*m3*q1_p*q2_p*sin(q3) + 8*I3_zz*L1^2*L2*L3*m1*m3*q2_p*q3_p*sin(q3) + 24*I3_zz*L1^2*L2*L3*m2*m3*q1_p*q3_p*sin(q3) + 24*I3_zz*L1^2*L2*L3*m2*m3*q2_p*q3_p*sin(q3) + 8*I2_zz*L1^2*L2*L3*m2*m3*q1_p*q2_p*sin(2*q2 + q3) - 8*I3_zz*L1^2*L2*L3*m2*m3*q1_p*q2_p*sin(2*q2 + q3) - 8*I3_zz*L1^2*L2*L3*m2*m3*q1_p*q3_p*sin(2*q2 + q3) - 8*I3_zz*L1^2*L2*L3*m2*m3*q2_p*q3_p*sin(2*q2 + q3)))/(64*I1_zz*I2_zz*I3_zz + 16*I2_zz*I3_zz*L1^2*m1 + 16*I1_zz*I3_zz*L2^2*m2 + 64*I2_zz*I3_zz*L1^2*m2 + 16*I1_zz*I2_zz*L3^2*m3 + 64*I1_zz*I3_zz*L2^2*m3 + 64*I2_zz*I3_zz*L1^2*m3 + 8*I3_zz*L1^2*L2^2*m2^2 + 8*I1_zz*L2^2*L3^2*m3^2 + 8*I2_zz*L1^2*L3^2*m3^2 + 32*I3_zz*L1^2*L2^2*m3^2 - 8*I2_zz*L1^2*L3^2*m3^2*cos(2*q2 + 2*q3) + 2*L1^2*L2^2*L3^2*m1*m3^2 + 6*L1^2*L2^2*L3^2*m2*m3^2 + 2*L1^2*L2^2*L3^2*m2^2*m3 + 4*I3_zz*L1^2*L2^2*m1*m2 + 4*I2_zz*L1^2*L3^2*m1*m3 + 16*I3_zz*L1^2*L2^2*m1*m3 + 4*I1_zz*L2^2*L3^2*m2*m3 + 16*I2_zz*L1^2*L3^2*m2*m3 + 48*I3_zz*L1^2*L2^2*m2*m3 - 8*I3_zz*L1^2*L2^2*m2^2*cos(2*q2) - 32*I3_zz*L1^2*L2^2*m3^2*cos(2*q2) - 8*I1_zz*L2^2*L3^2*m3^2*cos(2*q3) - 32*I3_zz*L1^2*L2^2*m2*m3*cos(2*q2) + L1^2*L2^2*L3^2*m1*m2*m3 - 2*L1^2*L2^2*L3^2*m1*m3^2*cos(2*q3) - 4*L1^2*L2^2*L3^2*m2*m3^2*cos(2*q2) - 2*L1^2*L2^2*L3^2*m2^2*m3*cos(2*q2) - 4*L1^2*L2^2*L3^2*m2*m3^2*cos(2*q3) + 2*L1^2*L2^2*L3^2*m2*m3^2*cos(2*q2 + 2*q3));
%     tau1_act = D1*q1_p + q3_pp*(I3_zz + (L3^2*m3)/4 + (L1*L3*m3*cos(q2 + q3))/2 + (L2*L3*m3*cos(q3))/2) + q1_pp*(I1_zz + I2_zz + I3_zz + (L1^2*m1)/4 + L1^2*m2 + L1^2*m3 + (L2^2*m2)/4 + L2^2*m3 + (L3^2*m3)/4 + L1*L3*m3*cos(q2 + q3) + L1*L2*m2*cos(q2) + 2*L1*L2*m3*cos(q2) + L2*L3*m3*cos(q3)) + (5*g*(7*L2*cos(q1 + q2) + 14*L1*cos(q1) + 2*L3*cos(q1 + q2 + q3)))/2 + q2_pp*(I2_zz + I3_zz + (L2^2*m2)/4 + L2^2*m3 + (L3^2*m3)/4 + (L1*L3*m3*cos(q2 + q3))/2 + (L1*L2*m2*cos(q2))/2 + L1*L2*m3*cos(q2) + L2*L3*m3*cos(q3)) - (L1*q2_p^2*(L3*m3*sin(q2 + q3) + L2*m2*sin(q2) + 2*L2*m3*sin(q2)))/2 - (L3*m3*q3_p^2*(L1*sin(q2 + q3) + L2*sin(q3)))/2 - L1*q1_p*q2_p*(L3*m3*sin(q2 + q3) + L2*m2*sin(q2) + 2*L2*m3*sin(q2)) - L3*m3*q1_p*q3_p*(L1*sin(q2 + q3) + L2*sin(q3)) - L3*m3*q2_p*q3_p*(L1*sin(q2 + q3) + L2*sin(q3));
%     tau2_act = D2*q2_p + I2_zz*q1_pp + I2_zz*q2_pp + I3_zz*q1_pp + I3_zz*q2_pp + I3_zz*q3_pp + 5*L3*g*cos(q1 + q2 + q3) + (35*L2*g*cos(q1 + q2))/2 + (L2^2*m2*q1_pp)/4 + (L2^2*m2*q2_pp)/4 + L2^2*m3*q1_pp + L2^2*m3*q2_pp + (L3^2*m3*q1_pp)/4 + (L3^2*m3*q2_pp)/4 + (L3^2*m3*q3_pp)/4 + (L1*L2*m2*q1_p^2*sin(q2))/2 + L1*L2*m3*q1_p^2*sin(q2) - (L2*L3*m3*q3_p^2*sin(q3))/2 + (L1*L3*m3*q1_pp*cos(q2 + q3))/2 + (L1*L2*m2*q1_pp*cos(q2))/2 + L1*L2*m3*q1_pp*cos(q2) + L2*L3*m3*q1_pp*cos(q3) + L2*L3*m3*q2_pp*cos(q3) + (L2*L3*m3*q3_pp*cos(q3))/2 + (L1*L3*m3*q1_p^2*sin(q2 + q3))/2 - L2*L3*m3*q1_p*q3_p*sin(q3) - L2*L3*m3*q2_p*q3_p*sin(q3);
%     tau3_act = (L3*m3*(L1*sin(q2 + q3) + L2*sin(q3))*q1_p^2)/2 + L2*L3*m3*sin(q3)*q1_p*q2_p + (L2*L3*m3*sin(q3)*q2_p^2)/2 + D3*q3_p + q2_pp*((m3*L3^2)/4 + (L2*m3*cos(q3)*L3)/2 + I3_zz) + q1_pp*(I3_zz + (L3^2*m3)/4 + (L1*L3*m3*cos(q2 + q3))/2 + (L2*L3*m3*cos(q3))/2) + q3_pp*((m3*L3^2)/4 + I3_zz) + 5*L3*g*cos(q1 + q2 + q3);
    output = [q1_p, q2_p, q3_p, q1_pp, q2_pp, q3_pp, tau1, tau2, tau3];
end

== matlab function project_bonus/q mux ==
  data: input input; q output; qp output
function [q, qp]  = q_mux(input)
    q1 = input(1);
    q2 = input(2);
    q3 = input(3);
    q1_p = input(4);
    q2_p = input(5);
    q3_p = input(6);
    q = [q1, q2, q3];
    qp = [q1_p, q2_p, q3_p];
end
